simulink model "Ex7"  (R2021b)
settings: Solver=VariableStepAuto  StartTime=0.0  StopTime=10.0  RelTol=1e-3
settings Model: Creator=benec  LastModifiedBy=benec

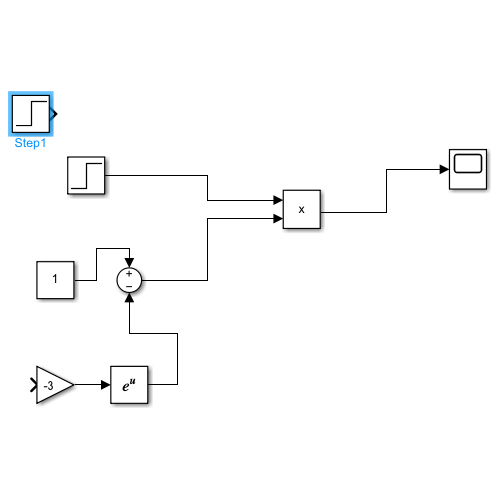
[thumbnail: Simulink's stored preview of the top-level diagram]
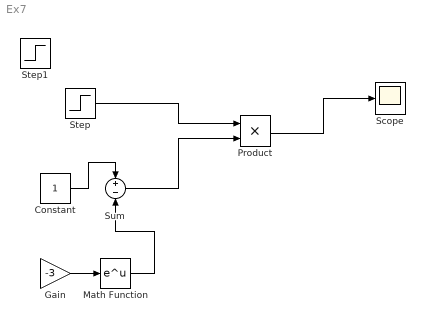
== system Ex7 ==
  Constant : Constant
  Gain : Gain  Gain=-3
  Math Function : Math  SaturateOnIntegerOverflow=on
  Product : Product
  Scope : Scope
  Step : Step  SampleTime=0
  Step1 : Step  Before=1  SampleTime=0
  Sum : Sum  Inputs=+-
  wires:
  Gain/1 -> Math Function/1
  Math Function/1 -> Sum/2
  Constant/1 -> Sum/1
  Sum/1 -> Product/2
  Step/1 -> Product/1
  Product/1 -> Scope/1
